simulink model "sampling_example"  (R2019b)
settings: Solver=VariableStepAuto  StartTime=0.0  StopTime=simTime  RelTol=1e-3
values from neighbouring files (symbols this model uses):
  delta = sym('delta', 'real')    [finite_compuability.m]    (also in init_comparison_sd.m = 0.1; sampling_comp.m)
  x0 = [0;0;0]    [init_comparison_sd.m]
settings Model: Creator=mohd-  LastModifiedBy=mohd-

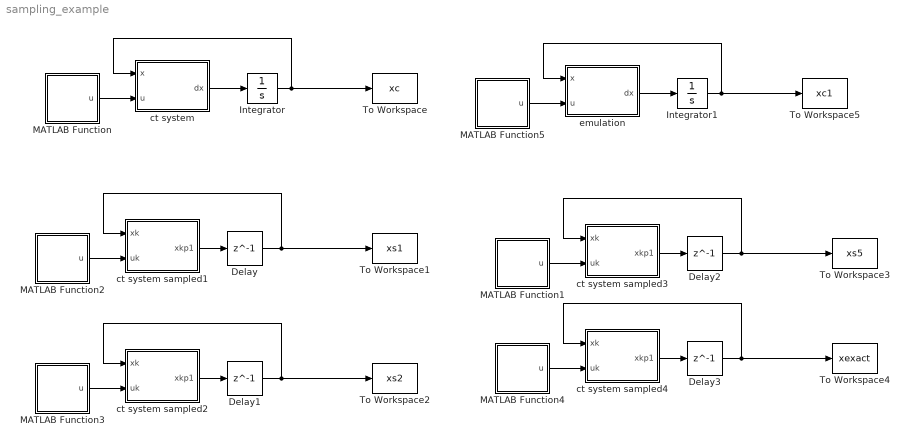
== system sampling_example ==
  Delay{,1..3} (4 alike) : Delay  DelayLength=1  InitialCondition=x0  SampleTime=delta
  Integrator : Integrator  InitialCondition=x0
  Integrator1 : Integrator  InitialCondition=x0
  MATLAB Function : MATLAB Function  TreatAsAtomicUnit=on
  MATLAB Function1 : MATLAB Function  TreatAsAtomicUnit=on  SystemSampleTime=delta
  MATLAB Function2 : MATLAB Function  TreatAsAtomicUnit=on  SystemSampleTime=delta
  MATLAB Function3 : MATLAB Function  TreatAsAtomicUnit=on  SystemSampleTime=delta
  MATLAB Function4 : MATLAB Function  TreatAsAtomicUnit=on  SystemSampleTime=delta
  MATLAB Function5 : MATLAB Function  TreatAsAtomicUnit=on  SystemSampleTime=delta
  To Workspace : ToWorkspace  VariableName=xc  SampleTime=10^-3
  To Workspace1 : ToWorkspace  VariableName=xs1  SampleTime=10^-3
  To Workspace2 : ToWorkspace  VariableName=xs2  SampleTime=10^-3
  To Workspace3 : ToWorkspace  VariableName=xs5  SampleTime=10^-3
  To Workspace4 : ToWorkspace  VariableName=xexact  SampleTime=10^-3
  To Workspace5 : ToWorkspace  VariableName=xc1  SampleTime=10^-3
  ct system : MATLAB Function  TreatAsAtomicUnit=on
  ct system sampled1 : MATLAB Function  TreatAsAtomicUnit=on
  ct system sampled2 : MATLAB Function  TreatAsAtomicUnit=on
  ct system sampled3 : MATLAB Function  TreatAsAtomicUnit=on
  ct system sampled4 : MATLAB Function  TreatAsAtomicUnit=on
  emulation : MATLAB Function  TreatAsAtomicUnit=on
  wires:
  ct system/1(dx) -> Integrator/1
  Integrator/1 -> To Workspace/1, ct system/1(x)
  MATLAB Function/1(u) -> ct system/2(u)
  MATLAB Function2/1(u) -> ct system sampled1/2(uk)
  ct system sampled1/1(xkp1) -> Delay/1
  Delay/1 -> To Workspace1/1, ct system sampled1/1(xk)
  ct system sampled2/1(xkp1) -> Delay1/1
  Delay1/1 -> To Workspace2/1, ct system sampled2/1(xk)
  MATLAB Function3/1(u) -> ct system sampled2/2(uk)
  ct system sampled3/1(xkp1) -> Delay2/1
  Delay2/1 -> To Workspace3/1, ct system sampled3/1(xk)
  MATLAB Function1/1(u) -> ct system sampled3/2(uk)
  Delay3/1 -> To Workspace4/1, ct system sampled4/1(xk)
  MATLAB Function4/1(u) -> ct system sampled4/2(uk)
  ct system sampled4/1(xkp1) -> Delay3/1
  MATLAB Function5/1(u) -> emulation/2(u)
  Integrator1/1 -> To Workspace5/1, emulation/1(x)
  emulation/1(dx) -> Integrator1/1

== matlab function sampling_example/MATLAB Function ==
  data: u output
function u = input()

u = [0.1;1];

== matlab function sampling_example/ct system ==
  data: x input; u input; dx output
function dx = dyn(x, u)


f  =  [0;0;0];
g   = [cos(x(3)) 0;
      sin(x(3)) 0;
      0         1];
dx = f + g*u;

== matlab function sampling_example/MATLAB Function1 ==
  data: u output
function u = input()

u = [0.1;1];

== matlab function sampling_example/ct system sampled3 ==
  data: xk input; uk input; xkp1 output; delta parameter
function xkp1 = dyn(xk, uk, delta)



f   =  [0;0;0];
g   = [cos(xk(3)) 0;
      sin(xk(3))  0;
      0           1];


x1 = xk(1); x2 = xk(2); x3 = xk(3); u1 = uk(1); u2 = uk(2);
xkp1  = [(u1*cos(x3)*delta^5*u2^4)/120 + (u1*sin(x3)*delta^4*u2^3)/24 - (u1*cos(x3)*delta^3*u2^2)/6 - (u1*sin(x3)*delta^2*u2)/2 + u1*cos(x3)*delta + x1;
        (u1*sin(x3)*delta^5*u2^4)/120 - (u1*cos(x3)*delta^4*u2^3)/24 - (u1*sin(x3)*delta^3*u2^2)/6 + (u1*cos(x3)*delta^2*u2)/2 + u1*sin(x3)*delta + x2;
                                                                                                                                        x3 + delta*u2];

== matlab function sampling_example/MATLAB Function2 ==
  data: u output
function u = input()

u = [0.1;1];

== matlab function sampling_example/ct system sampled1 ==
  data: xk input; uk input; xkp1 output; delta parameter
function xkp1 = dyn(xk, uk, delta)


f   =  [0;0;0];
g   = [cos(xk(3)) 0;
      sin(xk(3))  0;
      0           1];

xkp1 = xk + delta*(f + g*uk);

== matlab function sampling_example/MATLAB Function3 ==
  data: u output
function u = input()

u = [0.1;1];

== matlab function sampling_example/ct system sampled2 ==
  data: xk input; uk input; xkp1 output; delta parameter
function xkp1 = dyn(xk, uk, delta)


f   =  [0;0;0];
g   = [cos(xk(3)) 0;
      sin(xk(3))  0;
      0           1];

Lf_uLgId = [-sin(xk(3))*uk(1) 0; 
             cos(xk(3))*uk(1) 0;
             0                0];

         
xdd  = Lf_uLgId*uk;         
xkp1 = xk + delta*(f+g*uk) + delta^2/2* xdd;

== matlab function sampling_example/MATLAB Function4 ==
  data: u output
function u = input()

u = [0.1;1];

== matlab function sampling_example/ct system sampled4 ==
  data: xk input; uk input; xkp1 output; delta parameter
function xkp1 = dyn(xk, uk, delta)



f   =  [0;0;0];
g   = [cos(xk(3)) 0;
      sin(xk(3))  0;
      0           1];


x1 = xk(1); x2 = xk(2); x3 = xk(3); u1 = uk(1); u2 = uk(2);
xkp1 = xk + [ u1/u2*(sin(x3 + delta*u2) - sin(x3));
              u1/u2*(cos(x3) - cos(x3 +  delta*u2));
              delta*u2];

== matlab function sampling_example/MATLAB Function5 ==
  data: u output
function u = input()

u = [0.1;1];

== matlab function sampling_example/emulation ==
  data: x input; u input; dx output
function dx = dyn(x, u)


f  =  [0;0;0];
g   = [cos(x(3)) 0;
      sin(x(3)) 0;
      0         1];
dx = f + g*u;
